simulink model "DC_Grid_Sim_v1"  (R2023a)
settings: Solver=VariableStepAuto  StartTime=0.0  StopTime=1  RelTol=1e-3
model workspace (MATLAB code in the model file):
  | cables_temp=25;
undefined symbols (not defined in the file): AH, Cable_Temp, DiscIntNeverNeededParam, fsw, Ki, Kp, SOC0, Ts, Tsc
libraries: ee_lib x23, nesl_utility x15, fl_lib x12, eePwmGenerator x2, eeGeneralControl x1, slpidlib x1, batteryecm_lib x1
settings Model: Creator=duarte  LastModifiedBy=duarte

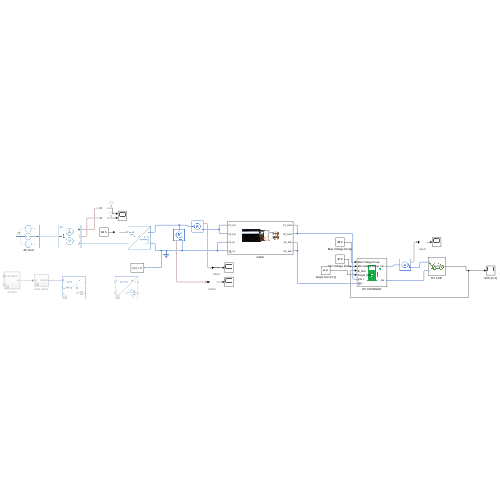
[thumbnail: Simulink's stored preview of the top-level diagram]
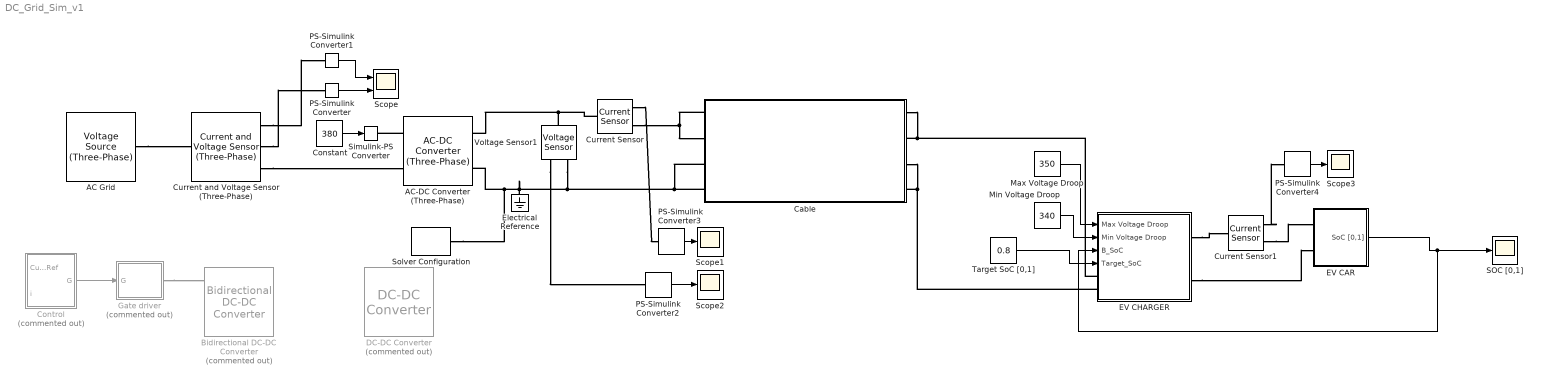
== system DC_Grid_Sim_v1 ==
  AC Grid : ee_lib/Sources/Voltage Source (Three-Phase)  vline_rms=sqrt(3) * 320 / sqrt(2) V  shift=0 deg  freq=50 Hz  impedance_option=1  SShortCircuit=1e6 A*V  XR=15  R=0.01 Ohm  L=3.97e-4 H  harmonic_option=1  harmonic_orders=[5, 7, 11, 13]  harmonic_ratios=[.1, .1, .1, .1]  G_parasitic=0 1/Ohm  I_specify=off  I_priority=None  I=[0, 0, 0] A  I_nominal_specify=off  I_nominal_unit=A  I_nominal_value=1
  AC-DC Converter (Three-Phase) : ee_lib/Semiconductors & Converters/Converters/AC-DC Converter (Three-Phase)  port_option=ee.enum.threePhasePort.composite  droop=0.5 V/A  Vdc_dynamics=ee.enum.converters.dynamics.yes  tauVdc=0.02 s  Vdc_ini=375 V  FRated=60 Hz  Vline_rms_min=200 V  tauVac=0.01 s  Vline_rms_ini=381 V  Vang_ini=0 deg  power_dynamics=ee.enum.converters.powerDynamics.no  tauP=0.01 s  P_ini=1e3 W  gmin=1e-6 S
      settings: InternalSimscapePortConfiguration="{\"Bottom\":[],\"Left\":[{\"id\":\"Vref\",\"label\":\"Vref\",\"type\":\"input\"},{\"id\":\"N\",\"label\":\"~\",\"type\":\"foundation.electrical.three_phase\"}],\"Right\":[{\"id\":\"p\",\"label\":\"+\",\"type\":\"foundation.electrical.electrical\"},{\"id\":\"n\",\"label\":\"-\",\"type\":\"foundation.electrical.electrical\"}],\"Top\":[]}"
  Bidirectional DC-DC Converter : ee_lib/Semiconductors & Converters/Converters/Bidirectional DC-DC Converter  Commented=on  device_type=ee.enum.converters.switchingdevice.ideal  Vf=0.8 V  Ron=0.001 Ohm  Rds=0.001 Ohm  Goff=1e-5 1/Ohm  Vth=6 V  Vgt=1 V  Vgt_off=-1 V  Ih=1 A  K=0  diode_param=ee.enum.converters.diode.nodynamics  diode_Vf=0.8 V  diode_Ron=0.001 Ohm  diode_Goff=1e-5 1/Ohm  diode_C=50 nF  diode_iRM=-235 A  diode_iF=300 A  diode_idot=-50 A/us  diode_trr_param=ee.enum.converters.diodetrr.trr_factor  diode_trr_factor=3  diode_trr=15 us  diode_Qrr=1500 s*uA  L=1e-6 H  Rl=0 Ohm  C1=1e-7 F  C2=1e-7 F  R1=1e-6 Ohm  R2=1e-6 Ohm  snubber_type=ee.enum.converters.snubber.exclude  Cs=1e-7 F  Rs=0.1 Ohm  iL_specify=off  iL_priority=High  iL=0 A  iL_nominal_specify=off  iL_nominal_unit=A  iL_nominal_value=1  vc1_specify=off  vc1_priority=High  vc1=0 V  vc1_nominal_specify=off  vc1_nominal_unit=V  vc1_nominal_value=1  vc2_specify=off  vc2_priority=High  vc2=0 V  vc2_nominal_specify=off  vc2_nominal_unit=V  vc2_nominal_value=1  device_type_hv=ee.enum.converters.switchingdevice.ideal  Vf_hv=0.8 V  Ron_hv=0.001 Ohm  Rds_hv=0.001 Ohm  Goff_hv=1e-5 1/Ohm  Vth_hv=6 V  Vgt_hv=1 V  Vgt_off_hv=-1 V  Ih_hv=1 A  device_type_lv=ee.enum.converters.switchingdevice.ideal  Vf_lv=0.8 V  Ron_lv=0.001 Ohm  Rds_lv=0.001 Ohm  Goff_lv=1e-5 1/Ohm  Vth_lv=6 V  Vgt_lv=1 V  Vgt_off_lv=-1 V  Ih_lv=1 A  T_L1=10 H  T_L2=0.1 H  T_k=0.9  snubber_type_hv=ee.enum.converters.snubber.exclude  Cs_hv=1e-7 F  Rs_hv=0.1 Ohm  snubber_type_lv=ee.enum.converters.snubber.exclude  Cs_lv=1e-7 F  Rs_lv=0.1 Ohm  iL1_specify=off  iL1_priority=High  iL1=0 A  iL1_nominal_specify=off  iL1_nominal_unit=A  iL1_nominal_value=1  iL2_specify=off  iL2_priority=High  iL2=0 A  iL2_nominal_specify=off  iL2_nominal_unit=A  iL2_nominal_value=1
      settings: InternalSimscapePortConfiguration="{\"Bottom\":[],\"Left\":[{\"id\":\"G\",\"label\":\"G\",\"type\":\"foundation.electrical.four_phase\"},{\"id\":\"p1\",\"label\":\"1+\",\"type\":\"foundation.electrical.electrical\"},{\"id\":\"n1\",\"label\":\"1-\",\"type\":\"foundation.electrical.electrical\"}],\"Right\":[{\"id\":\"p2\",\"label\":\"2+\",\"type\":\"foundation.electrical.electrical\"},{\"id\":\"n2\",\"label\":\"2-\",\"type\":\"foundation.electrical.electrical\"}],\"Top\":[]}"
  Cable : Subsystem  mask{CableLength=0.1, R20_km=1.91, Alpha=0.00403, L_km=0.3e-3, C_star_km=0.4e-6}
      mask prompts: CableLength "CableLength [km]"; R20_km "R20 [Ω/km] per conductor"; L_km "Inductance [H/km] per conductor"; C_star_km "Star Capacitance [F/km] per conductor"
      mask DialogControl ParameterGroupVar Prompt: Parametes
      mask DialogControl ParameterGroupVar_copy Prompt: Resistence
      mask Display: image('/home/duarte/Documents/INESC/EVDVGRID/Madeira_Port_DC_Grid_Sim/cabo-lsvav.png');
  Constant : Constant  Value=380
  Control : Subsystem  Commented=on
  Current Sensor : fl_lib/Electrical/Electrical Sensors/Current Sensor
  Current Sensor1 : fl_lib/Electrical/Electrical Sensors/Current Sensor
  Current and Voltage Sensor (Three-Phase) : ee_lib/Sensors & Transducers/Current and Voltage Sensor (Three-Phase)  vMeasurementType=ee.enum.vmeasurement.ll  outputUnit=ee.enum.unit.si  SRated=100e6 A*V  VRated=24e3 V  I_specify=off  I_priority=None  I=[0, 0, 0] A  I_nominal_specify=off  I_nominal_unit=A  I_nominal_value=1  V_specify=off  V_priority=None  V=[0, 0, 0] V  V_nominal_specify=off  V_nominal_unit=V  V_nominal_value=1
      settings: InternalSimscapePortConfiguration="{\"Bottom\":[],\"Left\":[{\"id\":\"N1\",\"label\":\"~1\",\"type\":\"foundation.electrical.three_phase\"}],\"Right\":[{\"id\":\"V_output\",\"label\":\"V\",\"type\":\"output\"},{\"id\":\"I_output\",\"label\":\"I\",\"type\":\"output\"},{\"id\":\"N2\",\"label\":\"~2\",\"type\":\"foundation.electrical.three_phase\"}],\"Top\":[]}"
  DC-DC Converter : ee_lib/Semiconductors & Converters/Converters/DC-DC Converter  Commented=on  Vref_option=ee.enum.converters.voltageref.internal  v_ref=10 V  P_rated=10 W  droop_enabled=true  droop_param=ee.enum.converters.droop.percent  droop=0.1 V/A  droop_percent=2  Vref_droop=10 V  reversible=ee.enum.converters.directionality.unidirectional  G_diode=1e-8 1/Ohm  P_fixed=1 W  losses_option=ee.enum.converters.lossesOption.proportionalToSquaredCurrent  eff_rated=80  tableOption=ee.enum.converters.lossTableOptionThermal.currentTemp  i_eff_vec=[-2, -1, 1, 2] A  v_eff_vec=[15, 30, 45] V  eff_vec=[66, 76, 80, 74]  eff_2D_table=[66, 66, 66; 76, 76, 76; 80, 80, 80; 74, 74, 74]  model_dynamics=ee.enum.converters.dynamics.no  tau=0.02 s  v_ini=10 V  v1_min=1 V  R1=1000 Ohm  R2=1000 Ohm  enable_fault=simscape.enum.onoff.off  fault_condition=ee.enum.faults.faultInputCondition.greaterThan  fault_threshold=0.5  T_eff_vec=[280, 300, 320] K  eff_3D_table=repmat([66; 76; 80; 74], 1, 3, 3)  thermal_mass=100 J/K  initial_temperature=298.15 K
      settings: InternalSimscapePortConfiguration="{\"Bottom\":[],\"Left\":[{\"id\":\"p1\",\"label\":\"1+\",\"type\":\"foundation.electrical.electrical\"},{\"id\":\"n1\",\"label\":\"1-\",\"type\":\"foundation.electrical.electrical\"}],\"Right\":[{\"id\":\"p2\",\"label\":\"2+\",\"type\":\"foundation.electrical.electrical\"},{\"id\":\"n2\",\"label\":\"2-\",\"type\":\"foundation.electrical.electrical\"}],\"Top\":[]}"
  EV CAR : Subsystem
      mask Display: image('$imagefile'); % Use "Edit Image" on toolstrip to change.
  EV CHARGER : Subsystem  mask{EvChargerPower_kW=11}
      mask prompts: EvChargerPower_kW "ChargerPower[kW]"
      mask Display: image('$imagefile'); % Use "Edit Image" on toolstrip to change.
  Electrical Reference : fl_lib/Electrical/Electrical Elements/Electrical Reference
  Gate driver : Subsystem  Commented=on
  Max Voltage Droop : Constant  Value=350  OutMin=[350]  OutMax=[380]
  Min Voltage Droop : Constant  Value=340  OutMin=[320]  OutMax=[350]
  PS-Simulink Converter{,1..4} (5 alike) : nesl_utility/PS-Simulink Converter  PhysicalDomain=network_engine_domain  SubClassName=ps_output  LeftPortType=input  RightPortType=output  PseudoPeriodic=off  Frequencies=[]  VectorFormat=inherit  Unit=inherit  AffineConversion=off
  SOC [0,1] : Scope
  Scope : Scope  NumInputPorts=2
  Scope1 : Scope
  Scope2 : Scope
  Scope3 : Scope
  Simulink-PS Converter : nesl_utility/Simulink-PS Converter  PhysicalDomain=network_engine_domain  SubClassName=ps_input  LeftPortType=input  RightPortType=output  PseudoPeriodic=off  Frequencies=[]  NoiseDistribution=none  NoiseParameters=[]  Unit=1  AffineConversion=off  FilteringAndDerivatives=provide  SimscapeFilterOrder=1  InputFilterTimeConstant=0.001  UdotUserProvided=0
  Solver Configuration : nesl_utility/Solver Configuration  PhysicalDomain=network_engine_domain  SubClassName=solver  LeftPortType=input  RightPortType=generic  Tones=[]  Harmonics=[]  SimulateNoise=off  Profile=off  UseLocalSampling=off  EnableSwitchedLinearOptims=on  FrequencyDomain=off  UseCCode=off  RelTol=0.001  AbsTol=0.001  MinStep=1e-09  ToWorkspace=off  RevertToSquareIcSolve=off  NumHomotopyIterations=100  PhasorMode=off  PhasorModeNumHarmonics=1  ConsistencySolver=NEWTON_XTOL_AFTER_FTOL  IndexReductionMethod=DerivativeReplacement  DoDC=on  ResidualTolerance=1e-09  ConsistencyTolSource=GLOBAL  ConsistencyAbsTol=0.001  ConsistencyRelTol=0.001  ConsistencyTolFactor=0.001  UseLocalSolver=on  LocalSolverChoice=NE_BACKWARD_EULER_ADVANCER  ResolveIndetEquations=on  FunctionEvalNumThread=1  LocalSolverSampleTime=100e-6  DoFixedCost=on  MaxNonlinIter=3  MaxModeIter=2  ComputeImpulses=off  ImpulseIterations=2  LinearAlgebra=auto  LinearAlgebraNumThread=0  EquationFormulation=NE_TIME_EF  DelaysMemoryBudget=1024  AutomaticFiltering=on  FilteringTimeConstant=0.001  PartitionStorageMethod=AS_NEEDED  PartitionMemoryBudget=1024  PartitionMethod=ROBUST
  Target SoC [0,1] : Constant  Value=0.8
  Voltage Sensor1 : fl_lib/Electrical/Electrical Sensors/Voltage Sensor
  wires:
  Control/1(G) -> Gate driver/1(G)
  Max Voltage Droop/1 -> EV CHARGER/1(Max Voltage Droop)
  Min Voltage Droop/1 -> EV CHARGER/2(Min Voltage Droop)
  EV CAR/1(SoC [0,1]) -> EV CHARGER/3(B_SoC), SOC [0,1]/1
  Target SoC [0,1]/1 -> EV CHARGER/4(Target_SoC)
  PS-Simulink Converter1/1 -> Scope/1
  PS-Simulink Converter/1 -> Scope/2
  Constant/1 -> Simulink-PS Converter/1
  PS-Simulink Converter3/1 -> Scope1/1
  PS-Simulink Converter2/1 -> Scope2/1
  PS-Simulink Converter4/1 -> Scope3/1
  connections:
  Cable/LConn4 -- Cable/LConn3 -- Voltage Sensor1/RConn2 -- Electrical Reference/LConn1 -- Solver Configuration/RConn1 -- AC-DC Converter (Three-Phase)/RConn2
  Voltage Sensor1/LConn1 -- AC-DC Converter (Three-Phase)/RConn1 -- Current Sensor/LConn1
  Gate driver/RConn1 -- Bidirectional DC-DC Converter/LConn1
  Cable/RConn1 -- EV CHARGER/LConn1 -- Cable/RConn2
  Cable/RConn3 -- EV CHARGER/LConn2 -- Cable/RConn4
  Current and Voltage Sensor (Three-Phase)/RConn3 -- AC-DC Converter (Three-Phase)/LConn2
  AC Grid/RConn1 -- Current and Voltage Sensor (Three-Phase)/LConn1
  Current and Voltage Sensor (Three-Phase)/RConn1 -- PS-Simulink Converter1/LConn1
  Current and Voltage Sensor (Three-Phase)/RConn2 -- PS-Simulink Converter/LConn1
  AC-DC Converter (Three-Phase)/LConn1 -- Simulink-PS Converter/RConn1
  EV CHARGER/RConn2 -- EV CAR/LConn2
  Voltage Sensor1/RConn1 -- PS-Simulink Converter2/LConn1
  Cable/LConn1 -- Current Sensor/RConn2 -- Cable/LConn2
  Current Sensor/RConn1 -- PS-Simulink Converter3/LConn1
  EV CHARGER/RConn1 -- Current Sensor1/LConn1
  Current Sensor1/RConn2 -- EV CAR/LConn1
  Current Sensor1/RConn1 -- PS-Simulink Converter4/LConn1

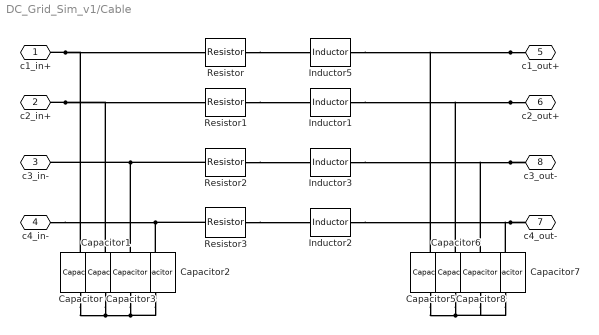
== system DC_Grid_Sim_v1/Cable ==
  Capacitor{,1..3,5..8} (8 alike) : ee_lib/Passive/Capacitor  cap_option=ee.enum.passive.capacitor.capOption.const  c=C_star_km * CableLength F  Cvec=[1e-05, 1e-06] F  Vvec=[0, 10] V  CV_table_symmetry=ee.enum.passive.capacitor.tableSymmetry.yes  f_vec=[1, 10] kHz  DFext_vec=[.8, 1.2]  enable_C_tol=ee.enum.toleranceApplication.none  averaging_period=0 s  C_tol=5  tol_distribution=ee.enum.toleranceDistribution.uniform  nSigma=4  r=1e-6 Ohm  g=0 1/Ohm  enable_operating_limits=ee.enum.enable.no  operating_limit_action=ee.enum.passive.reportOpLim.warn  max_working_voltage_range=[-25, 25] V  power_rating=1 W  enable_faults=ee.enum.enable.no  fault_action=simscape.enum.assert.action.none  Cscale_faulted=100  R_faulted=1e-3 Ohm  G_faulted=0 1/Ohm  tau_fault=1e-3 s  fault_trigger=ee.enum.faults.faultTrigger.temporal  t_fault=1 s  max_permissible_voltage_range=[-100, 100] V  t_fail_on_voltage=1 s  i_specify=off  i_priority=None  i=0 A  i_nominal_specify=off  i_nominal_unit=A  i_nominal_value=1  v_specify=off  v_priority=None  v=0 V  v_nominal_specify=off  v_nominal_unit=V  v_nominal_value=1  vc_specify=off  vc_priority=High  vc=0 V  vc_nominal_specify=off  vc_nominal_unit=V  vc_nominal_value=1
  Inductor{1..3,5} (4 alike) : ee_lib/Passive/Inductor  l=L_km*CableLength H  enable_L_tol=ee.enum.toleranceApplication.none  L_tol=20  tol_distribution=ee.enum.toleranceDistribution.uniform  nSigma=4  r=0 Ohm  g=1e-9 1/Ohm  enable_operating_limits=ee.enum.enable.no  operating_limit_action=ee.enum.passive.reportOpLim.warn  max_working_current=1 A  power_rating=1 W  enable_faults=ee.enum.enable.no  fault_action=simscape.enum.assert.action.none  lambdaPercent=50  k_faulted=0.9999  turnsShort=ee.enum.passive.inductor.turnsShortOption.no  openCct=ee.enum.enable.no  groundShort=ee.enum.passive.inductor.groundShortOption.no  groundShortG=0 1/Ohm  tau_fault=1e-3 s  fault_trigger=ee.enum.faults.faultTrigger.temporal  t_fault=1 s  max_permissible_voltage=100 V  n_fail_on_voltage=1  max_permissible_current=1 A  t_fail_on_current=1 s  i_L_specify=off  i_L_priority=High  i_L=0 A  i_L_nominal_specify=off  i_L_nominal_unit=A  i_L_nominal_value=1
  Resistor : ee_lib/Passive/Resistor  R=CableLength* R20_km * (1 + Alpha*(Cable_Temp - 20)) Ohm  enable_R_tol=ee.enum.toleranceApplication.none  R_tol=5  tol_distribution=ee.enum.toleranceDistribution.uniform  nSigma=4  enable_operating_limits=ee.enum.enable.no  operating_limit_action=ee.enum.passive.reportOpLim.warn  power_rating=1 W  max_working_voltage=100 V  enable_faults=ee.enum.enable.no  fault_action=simscape.enum.assert.action.none  R_faulted=inf Ohm  fault_trigger=ee.enum.faults.faultTrigger.temporal  t_fault=1 s  max_permissible_current=1 A  t_fail_on_current=1 s  noise_mode=ee.enum.sources.noise.Disabled  Tdevice=25 degC  sample_time=1e-3 s  repeatability=ee.enum.ic.repeatability.notRepeatable  user_seed=0  auto_seed=3890346746  power_derating_T1=70 degC  power_derating_T2=155 degC  operating_temperature_range_vec=[-50, 150] degC  alpha=3.93e-3 1/K  Tmeas=25 degC  thermal_mass=100 J/K  temperature_specify=off  temperature_priority=High  temperature=298.15 K  temperature_nominal_specify=off  temperature_nominal_unit=K  temperature_nominal_value=1
  Resistor1 : ee_lib/Passive/Resistor  R=CableLength* R20_km * (1 + Alpha*(Cable_Temp - 20)) Ohm  enable_R_tol=ee.enum.toleranceApplication.none  R_tol=5  tol_distribution=ee.enum.toleranceDistribution.uniform  nSigma=4  enable_operating_limits=ee.enum.enable.no  operating_limit_action=ee.enum.passive.reportOpLim.warn  power_rating=1 W  max_working_voltage=100 V  enable_faults=ee.enum.enable.no  fault_action=simscape.enum.assert.action.none  R_faulted=inf Ohm  fault_trigger=ee.enum.faults.faultTrigger.temporal  t_fault=1 s  max_permissible_current=1 A  t_fail_on_current=1 s  noise_mode=ee.enum.sources.noise.Disabled  Tdevice=25 degC  sample_time=1e-3 s  repeatability=ee.enum.ic.repeatability.notRepeatable  user_seed=0  auto_seed=545404223  power_derating_T1=70 degC  power_derating_T2=155 degC  operating_temperature_range_vec=[-50, 150] degC  alpha=3.93e-3 1/K  Tmeas=25 degC  thermal_mass=100 J/K  temperature_specify=off  temperature_priority=High  temperature=298.15 K  temperature_nominal_specify=off  temperature_nominal_unit=K  temperature_nominal_value=1
  Resistor2 : ee_lib/Passive/Resistor  R=CableLength* R20_km * (1 + Alpha*(Cable_Temp - 20)) Ohm  enable_R_tol=ee.enum.toleranceApplication.none  R_tol=5  tol_distribution=ee.enum.toleranceDistribution.uniform  nSigma=4  enable_operating_limits=ee.enum.enable.no  operating_limit_action=ee.enum.passive.reportOpLim.warn  power_rating=1 W  max_working_voltage=100 V  enable_faults=ee.enum.enable.no  fault_action=simscape.enum.assert.action.none  R_faulted=inf Ohm  fault_trigger=ee.enum.faults.faultTrigger.temporal  t_fault=1 s  max_permissible_current=1 A  t_fail_on_current=1 s  noise_mode=ee.enum.sources.noise.Disabled  Tdevice=25 degC  sample_time=1e-3 s  repeatability=ee.enum.ic.repeatability.notRepeatable  user_seed=0  auto_seed=3922919431  power_derating_T1=70 degC  power_derating_T2=155 degC  operating_temperature_range_vec=[-50, 150] degC  alpha=3.93e-3 1/K  Tmeas=25 degC  thermal_mass=100 J/K  temperature_specify=off  temperature_priority=High  temperature=298.15 K  temperature_nominal_specify=off  temperature_nominal_unit=K  temperature_nominal_value=1
  Resistor3 : ee_lib/Passive/Resistor  R=CableLength* R20_km * (1 + Alpha*(Cable_Temp - 20)) Ohm  enable_R_tol=ee.enum.toleranceApplication.none  R_tol=5  tol_distribution=ee.enum.toleranceDistribution.uniform  nSigma=4  enable_operating_limits=ee.enum.enable.no  operating_limit_action=ee.enum.passive.reportOpLim.warn  power_rating=1 W  max_working_voltage=100 V  enable_faults=ee.enum.enable.no  fault_action=simscape.enum.assert.action.none  R_faulted=inf Ohm  fault_trigger=ee.enum.faults.faultTrigger.temporal  t_fault=1 s  max_permissible_current=1 A  t_fail_on_current=1 s  noise_mode=ee.enum.sources.noise.Enabled  Tdevice=25 degC  sample_time=1e-3 s  repeatability=ee.enum.ic.repeatability.notRepeatable  user_seed=0  auto_seed=2715962282  power_derating_T1=70 degC  power_derating_T2=155 degC  operating_temperature_range_vec=[-50, 150] degC  alpha=3.93e-3 1/K  Tmeas=25 degC  thermal_mass=100 J/K  temperature_specify=off  temperature_priority=High  temperature=298.15 K  temperature_nominal_specify=off  temperature_nominal_unit=K  temperature_nominal_value=1
  c1_in+ : PMIOPort  Side=Left
  c2_in+ : PMIOPort  Port=2  Side=Left
  c3_in- : PMIOPort  Port=3  Side=Left
  c4_in- : PMIOPort  Port=4  Side=Left
  c1_out+ : PMIOPort  Port=5  Side=Right
  c2_out+ : PMIOPort  Port=6  Side=Right
  c4_out- : PMIOPort  Port=7  Side=Right
  c3_out- : PMIOPort  Port=8  Side=Right
  connections:
  c1_in+/RConn1 -- Resistor/LConn1 -- Capacitor/LConn1
  c1_out+/RConn1 -- Inductor5/RConn1 -- Capacitor5/LConn1
  c2_out+/RConn1 -- Inductor1/RConn1 -- Capacitor6/LConn1
  c2_in+/RConn1 -- Resistor1/LConn1 -- Capacitor1/LConn1
  c3_out-/RConn1 -- Inductor3/RConn1 -- Capacitor8/RConn1
  Capacitor3/RConn1 -- Resistor2/LConn1 -- c3_in-/RConn1
  c4_out-/RConn1 -- Inductor2/RConn1 -- Capacitor7/RConn1
  c4_in-/RConn1 -- Capacitor2/RConn1 -- Resistor3/LConn1
  Capacitor/RConn1 -- Capacitor2/LConn1 -- Capacitor3/LConn1 -- Capacitor1/RConn1
  Capacitor5/RConn1 -- Capacitor7/LConn1 -- Capacitor8/LConn1 -- Capacitor6/RConn1
  Resistor2/RConn1 -- Inductor3/LConn1
  Resistor3/RConn1 -- Inductor2/LConn1
  Resistor1/RConn1 -- Inductor1/LConn1
  Resistor/RConn1 -- Inductor5/LConn1

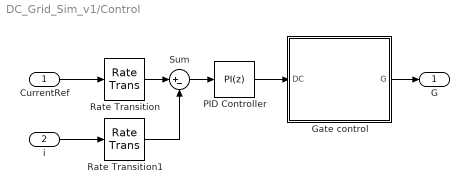
== system DC_Grid_Sim_v1/Control ==
  CurrentRef : Inport
  i : Inport  Port=2
  Gate control : Subsystem  Variant=on
  PID Controller : slpidlib/PID Controller  Controller=PI  Form=Parallel  TimeDomain=Discrete-time  UseExternalTs=off  SampleTime=Tsc  IntegratorMethod=Forward Euler  FilterMethod=Forward Euler  ControllerParametersSource=internal  P=Kp  I=Ki  UseKiTs=off  D=0  N=100  UseFilter=on  TunerSelectOption=Transfer Function Based (PID Tuner App)  InitialConditionSource=internal  InitialConditionForIntegrator=0  InitialConditionForFilter=0  DifferentiatorICPrevScaledInput=0  ExternalReset=none  TrackingMode=off  Kt=1  LimitOutput=on  SatLimitsSource=internal  UpperSaturationLimit=0.9  LowerSaturationLimit=0  LinearizeAsGain=on  AntiWindupMode=none  Kb=1  LimitIntegrator=off  UpperIntegratorSaturationLimit=inf  LowerIntegratorSaturationLimit=-inf  POutMin=[]  POutMax=[]  IOutMin=[]  IOutMax=[]  DOutMin=[]  DOutMax=[]  NOutMin=[]  NOutMax=[]  SumOutMin=[]  SumOutMax=[]  SaturationOutMin=[]  SaturationOutMax=[]  PParamMin=[]  PParamMax=[]  IParamMin=[]  IParamMax=[]  DParamMin=[]  DParamMax=[]  NParamMin=[]  NParamMax=[]  KbParamMin=[]  KbParamMax=[]  KtParamMin=[]  KtParamMax=[]  KbOutMin=[]  KbOutMax=[]  KtOutMin=[]  KtOutMax=[]  IntegratorOutMin=[]  IntegratorOutMax=[]  FilterOutMin=[]  FilterOutMax=[]  SumI1OutMin=[]  SumI1OutMax=[]  SumI2OutMin=[]  SumI2OutMax=[]  SumI3OutMin=[]  SumI3OutMax=[]  SumI4OutMin=[]  SumI4OutMax=[]  SumDOutMin=[]  SumDOutMax=[]  DifferentiatorOutMin=[]  DifferentiatorOutMax=[]  FilterDiffOutCoefMin=[]  FilterDiffOutCoefMax=[]  ReciprocalOutMin=[]  ReciprocalOutMax=[]  SumDenOutMin=[]  SumDenOutMax=[]  SumNumOutMin=[]  SumNumOutMax=[]  DivideOutMin=[]  DivideOutMax=[]  UdiffTsProdOutMin=[]  UdiffTsProdOutMax=[]  NTsProdOutMin=[]  NTsProdOutMax=[]  UintegralTsProdOutMin=[]  UintegralTsProdOutMax=[]  UngainTsProdOutMin=[]  UngainTsProdOutMax=[]  ClampingZeroOutDataTypeStr=Inherit: Inherit via back propagation  ClampingZeroOutMin=[]  ClampingZeroOutMax=[]  FilterDenConstantOutDataTypeStr=Inherit: Inherit via back propagation  FilterDenConstantOutMin=[]  FilterDenConstantOutMax=[]  PCopyOutDataTypeStr=Inherit: Inherit via back propagation  PCopyOutMin=[]  PCopyOutMax=[]  NCopyOutDataTypeStr=Inherit: Inherit via back propagation  NCopyOutMin=[]  NCopyOutMax=[]  IntegratorContinuousStateAttributes=''  IntegratorStateMustResolveToSignalObject=off  IntegratorRTWStateStorageClass=Auto  FilterContinuousStateAttributes=''  FilterStateMustResolveToSignalObject=off  FilterRTWStateStorageClass=Auto  ParallelPVariant=InternalParameters  IdealPVariant=Disabled  IVariant=InternalParameters  DVariant=Disabled  IntegratorVariant=Discrete  SatVariant=Enabled  AWVariant=Passthrough  PCopyVariant=Disabled  TRVariant=Disabled  FdbkBlocksVariant=Forward  IdealPFdbkVariant=Disabled  SatFdbkVariant=Disabled  DerivativeFilterVariant=Disabled  NVariant=Disabled  NCopyVariant=Disabled_SignalSpec  FilterICVariant=Disabled  IntegratorICVariant=InternalICs  ExternalResetVariant=Disabled  TRSumVariant=Passthrough  SumFdbkVariant=Disabled  SumVariant=Sum_PI  TsampFilterVariant=InternalTs  TsampNgainVariant=Passthrough  TsampIntegralVariant=Disabled_SignalSpec  ExternalSaturationOutDataTypeStr=Inherit: Same as second input
  Rate Transition : RateTransition
  Rate Transition1 : RateTransition
  Sum : Sum  Inputs=|+-
  G : Outport
  wires:
  CurrentRef/1 -> Rate Transition/1
  Sum/1 -> PID Controller/1
  i/1 -> Rate Transition1/1
  Gate control/1(G) -> G/1
  Rate Transition/1 -> Sum/1
  Rate Transition1/1 -> Sum/2
  PID Controller/1 -> Gate control/1(DC)

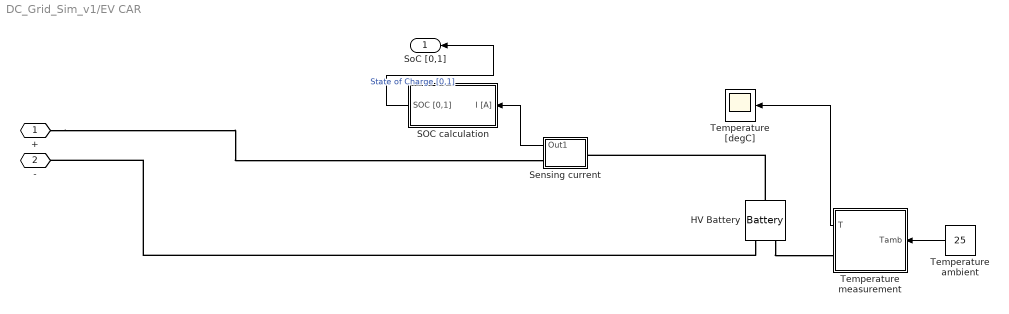
== system DC_Grid_Sim_v1/EV CAR ==
  HV Battery : batteryecm_lib/Battery  Vnom=Vnom V  prm_dir=1  R1_dis=2 Ohm  R1_ch=2 Ohm  R1=R0 Ohm  prm_AH=2  AH=AH hr*A  V1=V1 V  AH1=AH1 hr*A  prm_R2=1  R2=2000 Ohm  Tmeas=T1 degC  charge_measurement_port=simscape.enum.battery.enable.no  prm_dyn=simscape.enum.battery.prm_dyn.rc2  Rp1=R_RC1 Ohm  tau1=tau1 s  Rp2=R_RC2 Ohm  tau2=tau2 s  Rp3=0.005 Ohm  tau3=30 s  Rp4=0.005 Ohm  tau4=30 s  Rp5=0.005 Ohm  tau5=30 s  prm_fade=1  N_fade=100  AH_fade=45 hr*A  R1_fade=2.02 Ohm  R1_ch_fade=2.02 Ohm  V1_fade=10.35 V  prm_age=1  prm_age_OCV=1  OCV_age=0.9  SOC_age=60  Tmeas_age=298.15 K  delta_time_age_vec=[0] d  temperature_age_vec=[273] K  OCV_scaling_age=2.2134e6  OCV_offset_age=1.632e6  temp_exp_age=0.515833569 V  t_exp_age=0.75  Vnom_T2=Vnom_T2 V  R1_T2=R0_T2 Ohm  R1_T2_dis=2.2 Ohm  R1_T2_ch=2.2 Ohm  V1_T2=V1_T2 V  R2_T2=2200 Ohm  Rp1_T2=R_RC1_T2 Ohm  tau1_T2=tau1_T2 s  Rp2_T2=R_RC2_T2 Ohm  tau2_T2=tau2_T2 s  Rp3_T2=0.005 Ohm  tau3_T2=30 s  Rp4_T2=0.005 Ohm  tau4_T2=30 s  Rp5_T2=0.005 Ohm  tau5_T2=30 s  Tmeas2=T2 degC  thermal_port=simscape.enum.thermaleffects.model  thermal_mass=89400 J/K  i_specify=off  i_priority=None  i=0 A  i_nominal_specify=off  i_nominal_unit=A  i_nominal_value=1  v_specify=off  v_priority=None  v=0 V  v_nominal_specify=off  v_nominal_unit=V  v_nominal_value=1  charge_specify=on  charge_priority=High  charge="SOC0*AH  hr*A"  charge_nominal_specify=off  charge_nominal_unit=A*hr  charge_nominal_value=1  num_cycles_specify=off  num_cycles_priority=High  num_cycles=0  num_cycles_nominal_specify=off  num_cycles_nominal_unit=1  num_cycles_nominal_value=1  temperature_specify=on  temperature_priority=High  temperature=25 degC  temperature_nominal_specify=off  temperature_nominal_unit=K  temperature_nominal_value=1
      settings: InternalSimscapePortConfiguration="{\"Bottom\":[],\"Left\":[{\"id\":\"p\",\"label\":\"+\",\"type\":\"foundation.electrical.electrical\"}],\"Right\":[{\"id\":\"n\",\"label\":\"-\",\"type\":\"foundation.electrical.electrical\"},{\"id\":\"H\",\"label\":\"H\",\"type\":\"foundation.thermal.thermal\"}],\"Top\":[]}"
  SOC calculation : Subsystem
  Sensing current : Subsystem
      mask Display: disp('i')
  Temperature ambient : Constant  Value=25
  Temperature measurement : Subsystem
  Temperature [degC] : Scope
  + : PMIOPort  Side=Left
  - : PMIOPort  Port=2  Side=Left
  SoC [0,1] : Outport
  wires:
  Sensing current/1(Out1) -> SOC calculation/1(I [A])
  Temperature ambient/1 -> Temperature measurement/1(Tamb)
  SOC calculation/1(SOC [0,1]) -> SoC [0,1]/1  "State of Charge [0,1]"
  Temperature measurement/1(T) -> Temperature [degC]/1
  connections:
  HV Battery/LConn1 -- Sensing current/LConn1
  HV Battery/RConn2 -- Temperature measurement/RConn1
  HV Battery/RConn1 -- -/RConn1
  +/RConn1 -- Sensing current/RConn1

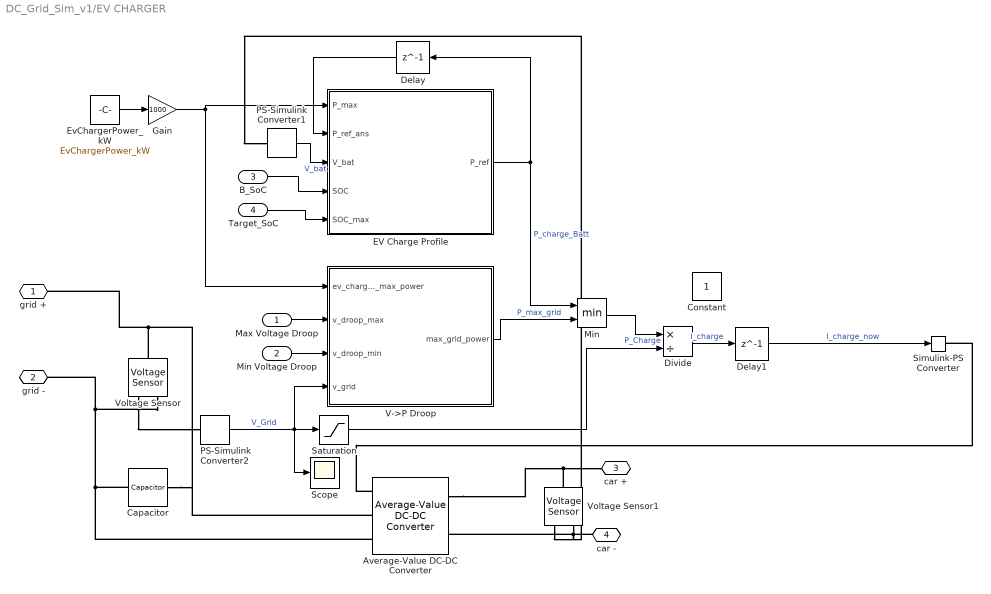
== system DC_Grid_Sim_v1/EV CHARGER ==
  Max Voltage Droop : Inport
  Min Voltage Droop : Inport  Port=2
  B_SoC : Inport  Port=3
  Target_SoC : Inport  Port=4
  Average-Value DC-DC Converter : ee_lib/Semiconductors & Converters/Converters/Average-Value DC-DC Converter  control_option=ee.enum.converters.controlinput.current  converter_type=ee.enum.converters.dcdctype.boost  efficiency_option=ee.enum.converters.efficiency.constant  efficiency_fixed=98  i_vec=[0, 2, 5] A  efficiency_vec=[90, 95, 98]
      settings: InternalSimscapePortConfiguration="{\"Bottom\":[],\"Left\":[{\"id\":\"Iref\",\"label\":\"Iref\",\"type\":\"input\"},{\"id\":\"p1\",\"label\":\"1+\",\"type\":\"foundation.electrical.electrical\"},{\"id\":\"n1\",\"label\":\"1-\",\"type\":\"foundation.electrical.electrical\"}],\"Right\":[{\"id\":\"p2\",\"label\":\"2+\",\"type\":\"foundation.electrical.electrical\"},{\"id\":\"n2\",\"label\":\"2-\",\"type\":\"foundation.electrical.electrical\"}],\"Top\":[]}"
  Capacitor : fl_lib/Electrical/Electrical Elements/Capacitor  c=1e-3 F  r=1e-2 Ohm  g=0 1/Ohm  i_specify=off  i_priority=None  i=0 A  i_nominal_specify=off  i_nominal_unit=A  i_nominal_value=1  v_specify=off  v_priority=None  v=0 V  v_nominal_specify=off  v_nominal_unit=V  v_nominal_value=1  vc_specify=off  vc_priority=High  vc=0 V  vc_nominal_specify=off  vc_nominal_unit=V  vc_nominal_value=1
  Constant : Constant
  Delay : Delay  DelayLength=1
  Delay1 : Delay  DelayLength=1
  Divide : Product  Inputs=*/
  EV Charge Profile : MATLAB Function  TreatAsAtomicUnit=on
  EvChargerPower_kW : Constant  Value=EvChargerPower_kW
  Gain : Gain  Gain=1000
  Min : MinMax  Inputs=2
  PS-Simulink Converter1 : nesl_utility/PS-Simulink Converter  PhysicalDomain=network_engine_domain  SubClassName=ps_output  LeftPortType=input  RightPortType=output  PseudoPeriodic=off  Frequencies=[]  VectorFormat=1-D array  Unit=V  AffineConversion=off
  PS-Simulink Converter2 : nesl_utility/PS-Simulink Converter  PhysicalDomain=network_engine_domain  SubClassName=ps_output  LeftPortType=input  RightPortType=output  PseudoPeriodic=off  Frequencies=[]  VectorFormat=1-D array  Unit=V  AffineConversion=off
  Saturation : Saturate  UpperLimit=inf  LowerLimit=320
  Scope : Scope
  Simulink-PS Converter : nesl_utility/Simulink-PS Converter  PhysicalDomain=network_engine_domain  SubClassName=ps_input  LeftPortType=input  RightPortType=output  PseudoPeriodic=off  Frequencies=[]  NoiseDistribution=none  NoiseParameters=[]  Unit=1  AffineConversion=off  FilteringAndDerivatives=provide  SimscapeFilterOrder=1  InputFilterTimeConstant=0.001  UdotUserProvided=0
  V->P Droop : MATLAB Function  TreatAsAtomicUnit=on
  Voltage Sensor : fl_lib/Electrical/Electrical Sensors/Voltage Sensor
  Voltage Sensor1 : fl_lib/Electrical/Electrical Sensors/Voltage Sensor
  grid + : PMIOPort  Side=Left
  grid - : PMIOPort  Port=2  Side=Left
  car + : PMIOPort  Port=3  Side=Right
  car - : PMIOPort  Port=4  Side=Right
  wires:
  Min Voltage Droop/1 -> V->P Droop/3(v_droop_min)
  Max Voltage Droop/1 -> V->P Droop/2(v_droop_max)
  EvChargerPower_kW/1 -> Gain/1
  V->P Droop/1(max_grid_power) -> Min/2  "P_max_grid"
  PS-Simulink Converter1/1 -> EV Charge Profile/3(V_bat)  "V_bat"
  B_SoC/1 -> EV Charge Profile/4(SOC)
  Target_SoC/1 -> EV Charge Profile/5(SOC_max)
  Gain/1 -> EV Charge Profile/1(P_max), V->P Droop/1(ev_charger_max_power)
  Saturation/1 -> Divide/2
  PS-Simulink Converter2/1 -> V->P Droop/4(v_grid), Scope/1, Saturation/1  "V_Grid"
  Min/1 -> Divide/1  "P_Charge"
  Divide/1 -> Delay1/1  "I_charge"
  EV Charge Profile/1(P_ref) -> Min/1, Delay/1  "P_charge_Batt"
  Delay/1 -> EV Charge Profile/2(P_ref_ans)
  Delay1/1 -> Simulink-PS Converter/1  "I_charge_now"
  connections:
  car -/RConn1 -- Voltage Sensor1/RConn2 -- Average-Value DC-DC Converter/RConn2
  Average-Value DC-DC Converter/LConn1 -- Simulink-PS Converter/RConn1
  Voltage Sensor/LConn1 -- Capacitor/LConn1 -- Average-Value DC-DC Converter/LConn2 -- grid +/RConn1
  Average-Value DC-DC Converter/RConn1 -- Voltage Sensor1/LConn1 -- car +/RConn1
  Average-Value DC-DC Converter/LConn3 -- Capacitor/RConn1 -- grid -/RConn1 -- Voltage Sensor/RConn2
  Voltage Sensor1/RConn1 -- PS-Simulink Converter1/LConn1
  Voltage Sensor/RConn1 -- PS-Simulink Converter2/LConn1

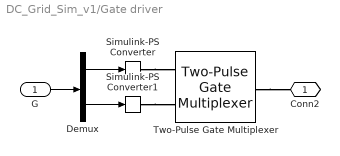
== system DC_Grid_Sim_v1/Gate driver ==
  G : Inport
  Demux : Demux  Outputs=2
  Simulink-PS Converter : nesl_utility/Simulink-PS Converter  PhysicalDomain=network_engine_domain  SubClassName=ps_input  LeftPortType=input  RightPortType=output  PseudoPeriodic=off  Frequencies=[]  NoiseDistribution=none  NoiseParameters=[]  Unit=1  AffineConversion=off  FilteringAndDerivatives=provide  SimscapeFilterOrder=1  InputFilterTimeConstant=0.001  UdotUserProvided=0
  Simulink-PS Converter1 : nesl_utility/Simulink-PS Converter  PhysicalDomain=network_engine_domain  SubClassName=ps_input  LeftPortType=input  RightPortType=output  PseudoPeriodic=off  Frequencies=[]  NoiseDistribution=none  NoiseParameters=[]  Unit=1  AffineConversion=off  FilteringAndDerivatives=provide  SimscapeFilterOrder=1  InputFilterTimeConstant=0.001  UdotUserProvided=0
  Two-Pulse Gate Multiplexer : ee_lib/Semiconductors & Converters/Converters/Two-Pulse Gate Multiplexer  port_option=ee.enum.controlport.ps
      settings: InternalSimscapePortConfiguration="{\"Bottom\":[],\"Left\":[{\"id\":\"G1_ps\",\"label\":\"G1\",\"type\":\"input\"},{\"id\":\"G2_ps\",\"label\":\"G2\",\"type\":\"input\"}],\"Right\":[{\"id\":\"p\",\"label\":\"G\",\"type\":\"foundation.electrical.four_phase\"}],\"Top\":[]}"
  Conn2 : PMIOPort  Side=Right
  wires:
  G/1 -> Demux/1
  Demux/1 -> Simulink-PS Converter/1
  Demux/2 -> Simulink-PS Converter1/1
  connections:
  Two-Pulse Gate Multiplexer/RConn1 -- Conn2/RConn1
  Simulink-PS Converter/RConn1 -- Two-Pulse Gate Multiplexer/LConn1
  Simulink-PS Converter1/RConn1 -- Two-Pulse Gate Multiplexer/LConn2

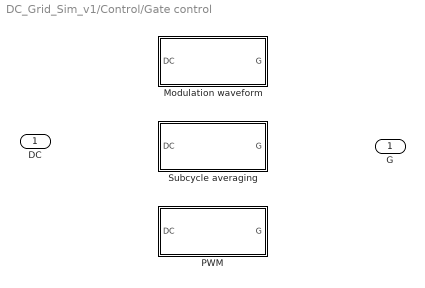
== system DC_Grid_Sim_v1/Control/Gate control ==
  DC : Inport
  Modulation waveform : Subsystem  VariantControl=gate_ctrl==1
  PWM : Subsystem  VariantControl=gate_ctrl==3
  Subcycle averaging : Subsystem  VariantControl=gate_ctrl==2
  G : Outport

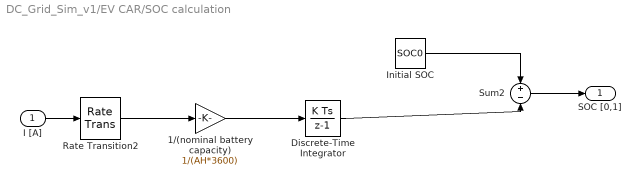
== system DC_Grid_Sim_v1/EV CAR/SOC calculation ==
  I [A] : Inport
  1/(nominal battery capacity) : Gain  Gain=1/(AH*3600)
  Discrete-Time Integrator : DiscreteIntegrator  SampleTime=-1  ICPrevOutput=DiscIntNeverNeededParam  ICPrevScaledInput=DiscIntNeverNeededParam
  Initial SOC : Constant  Value=SOC0
  Rate Transition2 : RateTransition
  Sum2 : Sum  Inputs=+-
  SOC [0,1] : Outport  VectorParamsAs1DForOutWhenUnconnected=off
  wires:
  I [A]/1 -> Rate Transition2/1
  Rate Transition2/1 -> 1/(nominal battery capacity)/1
  1/(nominal battery capacity)/1 -> Discrete-Time Integrator/1
  Initial SOC/1 -> Sum2/1
  Discrete-Time Integrator/1 -> Sum2/2
  Sum2/1 -> SOC [0,1]/1

== system DC_Grid_Sim_v1/EV CAR/Sensing current ==
  Current Sensor : fl_lib/Electrical/Electrical Sensors/Current Sensor
  PS-Simulink Converter2 : nesl_utility/PS-Simulink Converter  PhysicalDomain=network_engine_domain  SubClassName=ps_output  LeftPortType=input  RightPortType=output  PseudoPeriodic=off  Frequencies=[]  VectorFormat=1-D array  Unit=A  AffineConversion=off
  + : PMIOPort  Side=Left
  - : PMIOPort  Port=2  Side=Right
  Out1 : Outport  VectorParamsAs1DForOutWhenUnconnected=off
  wires:
  PS-Simulink Converter2/1 -> Out1/1
  connections:
  -/RConn1 -- Current Sensor/RConn2
  Current Sensor/RConn1 -- PS-Simulink Converter2/LConn1
  Current Sensor/LConn1 -- +/RConn1

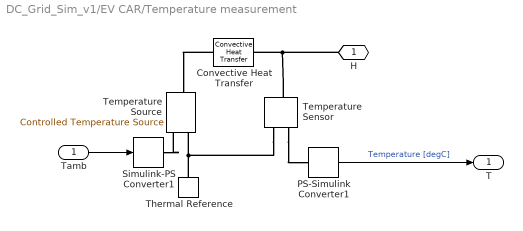
== system DC_Grid_Sim_v1/EV CAR/Temperature measurement ==
  Tamb : Inport
  Convective Heat Transfer : fl_lib/Thermal/Thermal Elements/Convective Heat Transfer  thermal_type=foundation.enum.constant_variable.constant  area=0.1 m^2  heat_tr_coeff=5 W/(m^2 * K)  min_heat_tr_coeff=1e-3 W/(K*m^2)  T_specify=off  T_priority=None  T=0 K  T_nominal_specify=off  T_nominal_unit=K  T_nominal_value=1  Q_specify=off  Q_priority=None  Q=0 J/s  Q_nominal_specify=off  Q_nominal_unit=J/s  Q_nominal_value=1
  PS-Simulink Converter1 : nesl_utility/PS-Simulink Converter  PhysicalDomain=network_engine_domain  SubClassName=ps_output  LeftPortType=input  RightPortType=output  PseudoPeriodic=off  Frequencies=[]  VectorFormat=1-D array  Unit=degC  AffineConversion=on
  Simulink-PS Converter1 : nesl_utility/Simulink-PS Converter  PhysicalDomain=network_engine_domain  SubClassName=ps_input  LeftPortType=input  RightPortType=output  PseudoPeriodic=off  Frequencies=[]  NoiseDistribution=none  NoiseParameters=[]  Unit=degC  AffineConversion=on  FilteringAndDerivatives=zero  SimscapeFilterOrder=1  InputFilterTimeConstant=0.001  UdotUserProvided=1
  Temperature Sensor : fl_lib/Thermal/Thermal Sensors/Temperature Sensor  temperature_measure=foundation.enum.MeasurementReference.difference
  Temperature Source : fl_lib/Thermal/Thermal Sources/Controlled Temperature Source
  Thermal Reference : fl_lib/Thermal/Thermal Elements/Thermal Reference
  H : PMIOPort  Side=Right
  T : Outport  VectorParamsAs1DForOutWhenUnconnected=off
  wires:
  Tamb/1 -> Simulink-PS Converter1/1
  PS-Simulink Converter1/1 -> T/1  "Temperature [degC]"
  connections:
  Convective Heat Transfer/RConn1 -- Temperature Source/LConn1
  Temperature Sensor/RConn2 -- PS-Simulink Converter1/LConn1
  Temperature Sensor/LConn1 -- H/RConn1 -- Convective Heat Transfer/LConn1
  Simulink-PS Converter1/RConn1 -- Temperature Source/RConn1
  Thermal Reference/LConn1 -- Temperature Sensor/RConn1 -- Temperature Source/RConn2

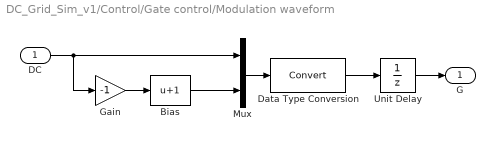
== system DC_Grid_Sim_v1/Control/Gate control/Modulation waveform ==
  DC : Inport
  Bias : Bias  Bias=1  SaturateOnIntegerOverflow=off
  Data Type Conversion : DataTypeConversion  SaturateOnIntegerOverflow=off  RndMeth=Floor
  Gain : Gain  Gain=-1
  Mux : Mux  Inputs=2
  Unit Delay : UnitDelay  SampleTime=-1  HasFrameUpgradeWarning=on
  G : Outport
  wires:
  DC/1 -> Gain/1, Mux/1
  Bias/1 -> Mux/2
  Gain/1 -> Bias/1
  Mux/1 -> Data Type Conversion/1
  Data Type Conversion/1 -> Unit Delay/1
  Unit Delay/1 -> G/1

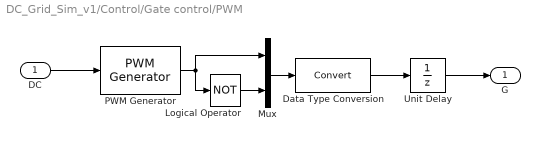
== system DC_Grid_Sim_v1/Control/Gate control/PWM ==
  DC : Inport
  Data Type Conversion : DataTypeConversion  SaturateOnIntegerOverflow=off  RndMeth=Floor
  Logical Operator : Logic  Operator=NOT  AllPortsSameDT=off  OutDataTypeStr=boolean
  Mux : Mux  Inputs=2
  PWM Generator : eePwmGenerator/PWM Generator  CarrCount=Up  Tper=1/fsw  Tdelay=0  Ts=Ts
  Unit Delay : UnitDelay  SampleTime=-1  HasFrameUpgradeWarning=on
  G : Outport
  wires:
  PWM Generator/1 -> Logical Operator/1, Mux/1
  DC/1 -> PWM Generator/1
  Mux/1 -> Data Type Conversion/1
  Logical Operator/1 -> Mux/2
  Data Type Conversion/1 -> Unit Delay/1
  Unit Delay/1 -> G/1

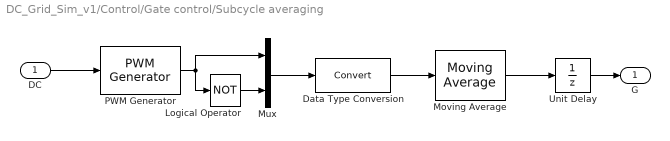
== system DC_Grid_Sim_v1/Control/Gate control/Subcycle averaging ==
  DC : Inport
  Data Type Conversion : DataTypeConversion  SaturateOnIntegerOverflow=off  RndMeth=Floor
  Logical Operator : Logic  Operator=NOT  AllPortsSameDT=off  OutDataTypeStr=boolean
  Moving Average : eeGeneralControl/Moving Average  VariantControl=Variant1  LabelModeActiveChoice=Discrete  f=40000  x0=0  BufferSize=8192  Ts=Ts
  Mux : Mux  Inputs=2
  PWM Generator : eePwmGenerator/PWM Generator  CarrCount=Up  Tper=1/fsw  Tdelay=0  Ts=Ts
  Unit Delay : UnitDelay  SampleTime=-1  HasFrameUpgradeWarning=on
  G : Outport
  wires:
  Mux/1 -> Data Type Conversion/1
  Data Type Conversion/1 -> Moving Average/1
  DC/1 -> PWM Generator/1
  PWM Generator/1 -> Logical Operator/1, Mux/1
  Logical Operator/1 -> Mux/2
  Moving Average/1 -> Unit Delay/1
  Unit Delay/1 -> G/1

== matlab function DC_Grid_Sim_v1/EV CHARGER/EV Charge Profile ==
  data: P_max input; P_ref_ans input; P_ref output; V_bat input; SOC input; SOC_max input
function P_ref = fcn(P_max, P_ref_ans, V_bat, SOC, SOC_max)
% EV charger power reference curve with voltage/SOC shaping
% and ramp-up / ramp-down limitation
%
% Inputs:
% P_max      - maximum charger power [W]
% P_ref_ans  - previous power reference [W]
% V_bat      - battery voltage [V]
% SOC        - battery state of charge [%]
% SOC_max    - maximum allowed SOC [%]
%
% Output:
% P_ref      - desired charger power after ramp limiter [W]

%% Voltage curve parameters

V_min  = 300;   % below this voltage, no charging
V_1    = 330;   % ramp-up region
V_2    = 360;   % full power starts
V_3    = 390;   % full power ends
V_4    = 410;   % ramp-down region
V_max  = 420;   % maximum battery voltage

%% SOC curve parameters

SOC_margin = 0.00;   % start reducing power 10% before SOC_max

%% Ramp limiter parameters

P_ramp_up   = 1000;   % max power increase per sample [W]
P_ramp_down = 2000;   % max power decrease per sample [W]

%% Safety limits

if P_max <= 0
    P_ref = 0;
    return;
end

if SOC >= SOC_max || V_bat >= V_max
    P_ref = 0;
    return;
end

%% Voltage factor k_v

% if V_bat <= V_min
%     k_v = 0;
% 
% elseif V_bat < V_1
%     % 0% -> 40%
%     x = (V_bat - V_min) / (V_1 - V_min);
%     k_v = 0.4 * smoothstep(x);
% 
% elseif V_bat < V_2
%     % 40% -> 100%
%     x = (V_bat - V_1) / (V_2 - V_1);
%     k_v = 0.4 + 0.6 * smoothstep(x);
% 
% elseif V_bat <= V_3
%     % Constant full power zone
%     k_v = 1;
% 
% elseif V_bat < V_4
%     % 100% -> 40%
%     x = (V_4 - V_bat) / (V_4 - V_3);
%     k_v = 0.4 + 0.6 * smoothstep(x);
% 
% elseif V_bat < V_max
%     % 40% -> 0%
%     x = (V_max - V_bat) / (V_max - V_4);
%     k_v = 0.4 * smoothstep(x);
% 
% else
%     k_v = 0;
% end

k_v = 1;

%% SOC factor k_soc

SOC_start = SOC_max - SOC_margin;

if SOC <= SOC_start
    k_soc = 1;

elseif SOC < SOC_max
    % Smooth ramp-down near SOC_max
    x = (SOC_max - SOC) / SOC_margin;
    k_soc = smoothstep(x);

else
    k_soc = 0;
end

%% Raw power command

k_total = min(k_v, k_soc);

P_cmd = P_max * k_total;

%% Ramp-up / Ramp-down limiter

delta_P = P_cmd - P_ref_ans;

if delta_P > P_ramp_up
    % Limit positive slope
    P_ref = P_ref_ans + P_ramp_up;

elseif delta_P < -P_ramp_down
    % Limit negative slope
    P_ref = P_ref_ans - P_ramp_down;

else
    % Within ramp limits
    P_ref = P_cmd;
end

%% Final protection

if P_ref > P_max
    P_ref = P_max;

elseif P_ref < 0
    P_ref = 0;
end

end


function y = smoothstep(x)
% Smooth transition from 0 to 1

if x < 0
    x = 0;

elseif x > 1
    x = 1;
end

y = x * x * (3 - 2 * x);

end

== matlab function DC_Grid_Sim_v1/EV CHARGER/V->P Droop ==
  data: ev_charger_max_power input; max_grid_power output; v_droop_max input; v_droop_min input; v_grid input
function max_grid_power = fcn(ev_charger_max_power, v_droop_max, v_droop_min, v_grid)

% Voltage-power droop control for DC/DC converter
% Low voltage  -> reduce grid/charger power
% High voltage -> allow maximum charger power

max_grid_power = ev_charger_max_power * ...
    (v_grid - v_droop_min) / (v_droop_max - v_droop_min);

% Saturation limits
if max_grid_power > ev_charger_max_power
    max_grid_power = ev_charger_max_power;
elseif max_grid_power < 0
    max_grid_power = 0;
end

end
